simulink model "Simulation_Fahrmodell_v3"  (R2023b)
settings: Solver=ode14x  StartTime=0.0  StopTime=600  FixedStep=0.005  RelTol=1e-3
values from neighbouring files (symbols this model uses):
  bat = bat.computePack()    [DoE_main.m]    (also in DoE_main_sensitivity.m)
  cp = cp.computeP4Map(val_P4, 0, val_P4_DM, 0, 0)    [DoE_main.m]    (also in DoE_main_sensitivity.m = cp.computeP4Map(P4, E2, P4_DM, E3, E4))
  gb = gb.computeShiftMaps()    [DoE_main.m]    (also in DoE_main_sensitivity.m)
  P4 = cfgNum(cfg, 'P4', 0)    [DoE_main_sensitivity.m]    (also in PowertrainConfig.m = 0)
  P4_DM = cfgNum(cfg, 'P4_DM', 0)    [DoE_main_sensitivity.m]    (also in PowertrainConfig.m = 0)
  pt = pt.setupHybrid()    [DoE_main.m]    (also in DoE_main_sensitivity.m)
  veh = VehicleConfig()    [DoE_main.m]    (also in DoE_main_sensitivity.m)
undefined symbols (not defined in the file or in its folder): cp_Zelle_JpkgK, Ice_derfacLoadDecrease_MAP, Ice_derfacLoadIncrease_MAP, Ice_n_axis, Ice_relLoadMax_CUR_n, Ice_relLoadMax_CUR_val, Ice_rl_axis_norm, seconds, SKO_STREET_CHAL, SKO_WHEEL_TYP_CHAL, slip_pacejka, T_init_degC, Track, TT_sliced, use_turbo_model, v_Fzg_init_kmph
libraries: nesl_utility x15, fl_lib x9
(part 3 of 6)

== system Simulation_Fahrmodell_v3/Vehicle Dynamics Model /Drivetrain/Reifenmodell1/Schlupfberechnung ==
  S_BUS_IST_Profil_a : Inport
  S_BUS_IST_Profil_v : Inport  Port=2
  AND : Logic  AllPortsSameDT=off  OutDataTypeStr=boolean
  Abs1 : Abs  SaturateOnIntegerOverflow=off
  Add1 : Sum
  Constant : Constant
  Constant1 : Constant
  Constant2 : Constant  Value=150
  Delay One Step : Delay  DelayLength=1
  Gain : Gain  Gain=3.6
  Gain1 : Gain  Gain=1/100
  GreaterThan1 : RelationalOperator  Operator=>  OutDataTypeStr=boolean  RndMeth=Simplest  InputSameDT=off
  GreaterThan2 : RelationalOperator  Operator=<=  OutDataTypeStr=boolean  RndMeth=Simplest  InputSameDT=off
  PS-Simulink Converter : nesl_utility/PS-Simulink Converter  PhysicalDomain=network_engine_domain  SubClassName=ps_output  LeftPortType=input  RightPortType=output  PseudoPeriodic=off  Frequencies=[]  VectorFormat=inherit  Unit=inherit  AffineConversion=off
  PS-Simulink Converter15 : nesl_utility/PS-Simulink Converter  PhysicalDomain=network_engine_domain  SubClassName=ps_output  LeftPortType=input  RightPortType=output  PseudoPeriodic=off  Frequencies=[]  VectorFormat=inherit  Unit=inherit  AffineConversion=off
  Schlupf als f(a[m/s^2]) : fl_lib/Physical Signals/Lookup Tables/PS Lookup Table (1D)  x=[0 2 4 6 8 10 12]  f=[4 5 6.5 8.5 9.25 10 10]  interp_method=simscape.enum.interpolation.smooth  extrap_method=simscape.enum.extrapolation.nearest
  Schlupf als f(v[km/h]) : fl_lib/Physical Signals/Lookup Tables/PS Lookup Table (1D)  x=[0 20 40 60 80 100 120]  f=[6 5.9 5.5 5 4.5 4.1 4]  interp_method=simscape.enum.interpolation.smooth  extrap_method=simscape.enum.extrapolation.nearest
  Scope1 : Scope  NumInputPorts=5
  Scope4 : Scope  NumInputPorts=2
  Simulink-PS Converter : nesl_utility/Simulink-PS Converter  PhysicalDomain=network_engine_domain  SubClassName=ps_input  LeftPortType=input  RightPortType=output  PseudoPeriodic=off  Frequencies=[]  NoiseDistribution=none  NoiseParameters=[]  Unit=1  AffineConversion=off  FilteringAndDerivatives=provide  SimscapeFilterOrder=1  InputFilterTimeConstant=0.001  UdotUserProvided=0
  Simulink-PS Converter3 : nesl_utility/Simulink-PS Converter  PhysicalDomain=network_engine_domain  SubClassName=ps_input  LeftPortType=input  RightPortType=output  PseudoPeriodic=off  Frequencies=[]  NoiseDistribution=none  NoiseParameters=[]  Unit=1  AffineConversion=off  FilteringAndDerivatives=provide  SimscapeFilterOrder=1  InputFilterTimeConstant=0.001  UdotUserProvided=0
  Solver Configuration1 : nesl_utility/Solver Configuration  PhysicalDomain=network_engine_domain  SubClassName=solver  LeftPortType=input  RightPortType=generic  Tones=[]  Harmonics=[]  SimulateNoise=off  Profile=off  UseLocalSampling=off  EnableSwitchedLinearOptims=on  FrequencyDomain=off  UseCCode=off  RelTol=0.001  AbsTol=0.001  MinStep=1e-09  ToWorkspace=off  RevertToSquareIcSolve=off  NumHomotopyIterations=100  PhasorMode=off  PhasorModeNumHarmonics=1  ConsistencySolver=NEWTON_FTOL  CanonicalOrdering=UNORDERED  OptimizeIntermediates=UNOPTIMIZED  IndexReductionMethod=DerivativeReplacement  DoDC=off  ResidualTolerance=1e-09  ConsistencyTolSource=GLOBAL  ConsistencyAbsTol=0.001  ConsistencyRelTol=0.001  ConsistencyTolFactor=0.001  UseLocalSolver=off  LocalSolverChoice=NE_BACKWARD_EULER_ADVANCER  ResolveIndetEquations=on  FunctionEvalNumThread=1  LocalSolverSampleTime=0.001  DoFixedCost=off  MaxNonlinIter=3  MaxModeIter=2  ComputeImpulses=off  ImpulseIterations=2  LinearAlgebra=auto  LinearAlgebraNumThread=0  EquationFormulation=NE_TIME_EF  DelaysMemoryBudget=1024  AutomaticFiltering=on  FilteringTimeConstant=0.001  PartitionStorageMethod=AS_NEEDED  PartitionMemoryBudget=1024  PartitionMethod=ROBUST  MultibodyUseLocalSolver=off  MultibodyLocalSolverChoice=ODE1  MultibodyLocalSolverSampleTime=0.001
  Solver Configuration2 : nesl_utility/Solver Configuration  PhysicalDomain=network_engine_domain  SubClassName=solver  LeftPortType=input  RightPortType=generic  Tones=[]  Harmonics=[]  SimulateNoise=off  Profile=off  UseLocalSampling=off  EnableSwitchedLinearOptims=on  FrequencyDomain=off  UseCCode=off  RelTol=0.001  AbsTol=0.001  MinStep=1e-09  ToWorkspace=off  RevertToSquareIcSolve=off  NumHomotopyIterations=100  PhasorMode=off  PhasorModeNumHarmonics=1  ConsistencySolver=NEWTON_FTOL  CanonicalOrdering=UNORDERED  OptimizeIntermediates=UNOPTIMIZED  IndexReductionMethod=DerivativeReplacement  DoDC=off  ResidualTolerance=1e-09  ConsistencyTolSource=GLOBAL  ConsistencyAbsTol=0.001  ConsistencyRelTol=0.001  ConsistencyTolFactor=0.001  UseLocalSolver=off  LocalSolverChoice=NE_BACKWARD_EULER_ADVANCER  ResolveIndetEquations=on  FunctionEvalNumThread=1  LocalSolverSampleTime=0.001  DoFixedCost=off  MaxNonlinIter=3  MaxModeIter=2  ComputeImpulses=off  ImpulseIterations=2  LinearAlgebra=auto  LinearAlgebraNumThread=0  EquationFormulation=NE_TIME_EF  DelaysMemoryBudget=1024  AutomaticFiltering=on  FilteringTimeConstant=0.001  PartitionStorageMethod=AS_NEEDED  PartitionMemoryBudget=1024  PartitionMethod=ROBUST  MultibodyUseLocalSolver=off  MultibodyLocalSolverChoice=ODE1  MultibodyLocalSolverSampleTime=0.001
  Switch1 : Switch  Criteria=u2 > Threshold  SaturateOnIntegerOverflow=off  InputSameDT=off
  s max (%) : Outport
  s_fakt : Outport  Port=2
  wires:
  S_BUS_IST_Profil_a/1 -> Delay One Step/1
  GreaterThan1/1 -> AND/1  "abs(a) > 1 m/s^2"
  Constant1/1 -> GreaterThan1/2
  S_BUS_IST_Profil_v/1 -> Gain/1
  PS-Simulink Converter15/1 -> Scope1/2, Switch1/3  "s (v)"
  Gain1/1 -> Add1/1
  GreaterThan2/1 -> AND/2  "v <= 150 km/h"
  Delay One Step/1 -> Scope4/1, Abs1/1, Simulink-PS Converter/1
  Constant/1 -> Add1/2
  PS-Simulink Converter/1 -> Switch1/1, Scope1/1  "S a)"
  Gain/1 -> Simulink-PS Converter3/1, GreaterThan2/1  "v (km/h)"
  Add1/1 -> Scope1/5, s_fakt/1  "s_fakt"
  AND/1 -> Scope1/3, Switch1/2  "beide Bedingungen erfüllt"
  Switch1/1 -> Scope1/4, s max (%)/1, Gain1/1  "s max (%)"
  Constant2/1 -> GreaterThan2/2
  Abs1/1 -> GreaterThan1/1, Scope4/2
  connections:
  Schlupf als f(a[m/s^2])/LConn1 -- Solver Configuration1/RConn1 -- Simulink-PS Converter/RConn1
  PS-Simulink Converter/LConn1 -- Schlupf als f(a[m/s^2])/RConn1
  Simulink-PS Converter3/RConn1 -- Solver Configuration2/RConn1 -- Schlupf als f(v[km/h])/LConn1
  Schlupf als f(v[km/h])/RConn1 -- PS-Simulink Converter15/LConn1

== system Simulation_Fahrmodell_v3/Vehicle Dynamics Model /Driving Resistance/Subsystem/Fahrwiderstand1 ==
  note: Kraftfahrtechnisches Taschenbuch | SpringerLink
  note: Kraftfahrtechnisches Handbuch - Bosch 2024
  note: Massenfaktor: Multiplikationsfaktor zur Masse abh. Hubraum
  note: Luftwiderstand
  note: Geschwindigkeitswiderstand
  note: Rollwiderstand
  note: Steigungswiderstand
  X_BUS_CHAL : Inport
  BUS_STEIGUNG : Inport  Port=2
  F_x_N : Inport  Port=3
  Add : Sum  Inputs=++++
  Bus Selector1 : BusSelector  OutputSignals=S_BUS_EIG_RoWi_CHAL,S_BUS_EIG_GEW_CHAL,S_BUS_EIG_A_CHAL,S_BUS_EIG_Cw_CHAL,S_BUS_EIG_v_Bwert_CHAL
  Bus Selector4 : BusSelector  OutputSignals=M_BUS_EIG_CHAL
  Divide : Product  Inputs=*/
  Erdbeschleunigung : Gain  Gain=9.81
  Gain : Gain  Gain=0.5
  Gain{1..5} (5 alike) : Gain
  Integrator : Integrator  InitialCondition=0.01
  MATLAB Function : MATLAB Function  TreatAsAtomicUnit=on
  MATLAB Function1 : MATLAB Function  TreatAsAtomicUnit=on
  Math Function : Math  Operator=square
  Mux1 : Mux  Inputs=2
  Mux2 : Mux  Inputs=5
  Product : Product
  Product1 : Product  Inputs=5
  Product2 : Product
  Product8 : Product
  Roh Luft : Constant  Value=1.23
  Scope : Scope  NumInputPorts=2
  Scope2 : Scope  NumInputPorts=2
  Sum : Sum  Inputs=-+
  v : Outport
  wires:
  Bus Selector1/1 -> Gain1/1  "<S_BUS_EIG_RoWi_CHAL>"
  MATLAB Function/1(y) -> Product1/5  "cosd(alpha)"
  Math Function/1 -> Product1/4  "v ^ 2"
  MATLAB Function1/1(y) -> Product2/2  "sind(alpha)"
  BUS_STEIGUNG/1 -> MATLAB Function1/1(u), MATLAB Function/1(u)  "alpha"
  Bus Selector1/2 -> Gain2/1  "<S_BUS_EIG_GEW_CHAL>"
  Bus Selector1/3 -> Gain3/1  "<S_BUS_EIG_A_CHAL>"
  Erdbeschleunigung/1 -> Product2/1, Product/2  "m * g"
  Roh Luft/1 -> Gain/1  "rho"
  Product2/1 -> Add/4, Scope/1, Mux2/4  "Steigungswiderstand (N)"
  Integrator/1 -> v/1, Product8/2, Math Function/1  "v"
  Add/1 -> Scope/2, Mux1/2, Sum/1  "S_BUS_FLST_Wrls (N)"
  Mux2/1 -> Scope2/1
  Bus Selector1/5 -> Gain5/1  "<S_BUS_EIG_v_Bwert_CHAL>"
  Mux1/1 -> Scope2/2
  Bus Selector1/4 -> Gain4/1  "<S_BUS_EIG_Cw_CHAL>"
  Product1/1 -> Add/2, Mux2/2  "Luftwiderstand (N)"
  Product/1 -> Add/1, Mux2/1  "Rollwiderstand (N)"
  Gain/1 -> Product1/2  "0,5 * rho"
  Product8/1 -> Add/3, Mux2/3  "Geschwindigkeitswiderstand (N)"
  Bus Selector4/1 -> Bus Selector1/1  "<M_BUS_EIG_CHAL>"
  X_BUS_CHAL/1 -> Bus Selector4/1
  Gain1/1 -> Product/1  "f_R"
  Gain2/1 -> Erdbeschleunigung/1, Divide/2  "m"
  Gain3/1 -> Product1/1  "A"
  Gain4/1 -> Product1/3  "Cw"
  Gain5/1 -> Product8/1  "f_v"
  F_x_N/1 -> Sum/2  "F_x_N"
  Sum/1 -> Divide/1
  Divide/1 -> Integrator/1

== system Simulation_Fahrmodell_v3/Vehicle Dynamics Model /Drivetrain/Axle Load and Torque Distribution /Drive Topology Axle Load Distributor /Front Axle Load Calculator  ==
  M_Nm : Inport
  Achslast HA [%] : Inport  Port=2
  Display : Display
  Display1 : Display
  Display2 : Display
  Gain : Gain  Gain=0.01
  Radlast HA : Product
  Radlast HA [Nm] : Outport
  wires:
  Achslast HA [%]/1 -> Display/1, Gain/1
  M_Nm/1 -> Radlast HA/1
  Gain/1 -> Display1/1, Radlast HA/2
  Radlast HA/1 -> Display2/1, Radlast HA [Nm]/1

== system Simulation_Fahrmodell_v3/Vehicle Dynamics Model /Drivetrain/Axle Load and Torque Distribution /Drive Topology Axle Load Distributor /P4 AWD or AWD ==
  M_VA_Nm IN : Inport
  In3 : Inport  Port=2
  In2 : Inport  Port=3
  Switch : Switch  Criteria=u2 > Threshold  SaturateOnIntegerOverflow=off  InputSameDT=off
  Out1 : Outport
  wires:
  In3/1 -> Switch/3
  Switch/1 -> Out1/1
  M_VA_Nm IN/1 -> Switch/1
  In2/1 -> Switch/2

== system Simulation_Fahrmodell_v3/Vehicle Dynamics Model /Drivetrain/Axle Load and Torque Distribution /Drive Topology Axle Load Distributor /P4 AWD or AWD1 ==
  In2 : Inport
  M_VA_Nm IN : Inport  Port=2
  In3 : Inport  Port=3
  Switch : Switch  Criteria=u2 > Threshold  SaturateOnIntegerOverflow=off  InputSameDT=off
  Out1 : Outport
  wires:
  In2/1 -> Switch/2
  M_VA_Nm IN/1 -> Switch/1
  Switch/1 -> Out1/1
  In3/1 -> Switch/3

== system Simulation_Fahrmodell_v3/Vehicle Dynamics Model /Drivetrain/Axle Load and Torque Distribution /Drive Topology Axle Load Distributor /Rear Axle Load Calculator  ==
  M_Nm : Inport
  Achslast VA [%] : Inport  Port=2
  Gain : Gain  Gain=0.01
  Radlast VA : Product
  Radlast VA [Nm] : Outport
  wires:
  Achslast VA [%]/1 -> Gain/1
  M_Nm/1 -> Radlast VA/1
  Radlast VA/1 -> Radlast VA [Nm]/1
  Gain/1 -> Radlast VA/2

== system Simulation_Fahrmodell_v3/Vehicle Dynamics Model /Drivetrain/GETRIEBE auswahl VK, EV/Transmission Selector/ EV Single-Speed ==
  n_mot_Upmin : Inport
  i_AG : Inport  Port=2
  "Gaspedalposition [0, 1]" : Inport  Port=3
  Constant : Constant  Value=gb.i_GET_EV
  "GET -> AG" : Product
  Terminator : Terminator
  Terminator1 : Terminator
  i_GES : Outport
  i_GES_delay : Outport  Port=2
  wires:
  "GET -> AG"/1 -> i_GES_delay/1, i_GES/1  "i_GES"
  Constant/1 -> "GET -> AG"/2
  i_AG/1 -> "GET -> AG"/1  "i_AG"
  n_mot_Upmin/1 -> Terminator/1
  "Gaspedalposition [0, 1]"/1 -> Terminator1/1

== system Simulation_Fahrmodell_v3/Vehicle Dynamics Model /Drivetrain/GETRIEBE auswahl VK, EV/Transmission Selector/ICE Multi-Speed ==
  note: Determination of minimum and maximum speed depending on accelerator pedal position and actual gear
  n_mot_Upmin : Inport
  i_AG : Inport  Port=2
  "Gaspedalposition [0, 1]" : Inport  Port=3
  Aktueller Gang : Gain
  Begrenzung Gang : Saturate  UpperLimit=10  LowerLimit=1
  Bus Creator : BusCreator  Inputs=3
  Delay Aktueller Gang Init: 1 : Delay  DelayLength=1  InitialCondition=1
  Delay Aktueller Gang Init: 2 : Delay  DelayLength=1  InitialConditionSource=Input port  InitialCondition=1
      settings: InputPortMap=u0,p4
  Ermittlung min und max Drehzahl abh. Gaspedalposition und Ist-Gang : Subsystem
  "GET -> AG" : Product
  Gain1 : Gain
  "Gang -> i_GET Generic 1" : Lookup_n-D  NumberOfTableDimensions=1  BreakpointsForDimension1=[1:1:gb.No_Gears]  Table=gb.Gear_Ratio  InternalRulePriority=Speed  RndMeth=Simplest
  Init: i_GES(1) Generic 1 : Constant  Value=5*3.204
  Scope : Scope  NumInputPorts=3
  Simulation Doppelkupplung (Gangwechsel ohne Zugkraftunterbrechung) orig2 : Subsystem
  Subsystem1 : Subsystem
  i_GES : Outport
  i_GES_delay : Outport  Port=2
  wires:
  Subsystem1/1(Current_Gear) -> Begrenzung Gang/1
  Init: i_GES(1) Generic 1/1 -> Delay Aktueller Gang Init: 2/2
  Ermittlung min und max Drehzahl abh. Gaspedalposition und Ist-Gang/2(n_min_Upmin) -> Subsystem1/3(downshift), Bus Creator/2
  Bus Creator/1 -> Scope/1
  Ermittlung min und max Drehzahl abh. Gaspedalposition und Ist-Gang/1(n_max_Upmin) -> Subsystem1/2(upshift), Bus Creator/3
  Gain1/1 -> "GET -> AG"/1  "i_AG"
  "Gang -> i_GET Generic 1"/1 -> "GET -> AG"/2
  "Gaspedalposition [0, 1]"/1 -> Ermittlung min und max Drehzahl abh. Gaspedalposition und Ist-Gang/1(Gaspedalposition)
  Simulation Doppelkupplung (Gangwechsel ohne Zugkraftunterbrechung) orig2/1(i_GET DKG) -> i_GES/1, Delay Aktueller Gang Init: 2/1, Scope/2
  n_mot_Upmin/1 -> Subsystem1/1(Current rpm), Bus Creator/1  "n_mot_Upmin"
  Begrenzung Gang/1 -> Delay Aktueller Gang Init: 1/1, Aktueller Gang/1
  Delay Aktueller Gang Init: 1/1 -> Ermittlung min und max Drehzahl abh. Gaspedalposition und Ist-Gang/2(Gang)
  i_AG/1 -> Gain1/1
  Aktueller Gang/1 -> "Gang -> i_GET Generic 1"/1, Simulation Doppelkupplung (Gangwechsel ohne Zugkraftunterbrechung) orig2/2(GANG), Scope/3  "GANG"
  "GET -> AG"/1 -> Simulation Doppelkupplung (Gangwechsel ohne Zugkraftunterbrechung) orig2/1(i_GET)  "i_GES"
  Delay Aktueller Gang Init: 2/1 -> i_GES_delay/1

== system Simulation_Fahrmodell_v3/Vehicle Dynamics Model /Drivetrain/Operating Strategy 1.1/EMs Priority (Ep)/SOC LIMIT ==
  tq_wheel_ICE_des_Ep : Inport
  SOC : Inport  Port=2
  tq_wheel_Elec_des_Ep : Inport  Port=3
  Add : Sum
  Constant : Constant  Value=0
  Ep_SOC Limit : Constant  Value=20
  Relational Operator : RelationalOperator  Operator=>  OutDataTypeStr=boolean  RndMeth=Simplest  InputSameDT=off
  Switch : Switch  Criteria=u2 > Threshold  SaturateOnIntegerOverflow=off  InputSameDT=off
  Switch1 : Switch  Criteria=u2 > Threshold  SaturateOnIntegerOverflow=off  InputSameDT=off
  "tq_wheel_ICE_des_Ep " : Outport
  "tq_wheel_Elec_des_Ep " : Outport  Port=2
  wires:
  Ep_SOC Limit/1 -> Relational Operator/2
  Relational Operator/1 -> Switch1/2, Switch/2
  tq_wheel_Elec_des_Ep/1 -> Switch1/1, Add/2
  Switch1/1 -> "tq_wheel_Elec_des_Ep "/1
  SOC/1 -> Relational Operator/1
  Constant/1 -> Switch1/3
  tq_wheel_ICE_des_Ep/1 -> Add/1, Switch/1
  Switch/1 -> "tq_wheel_ICE_des_Ep "/1
  Add/1 -> Switch/3

== system Simulation_Fahrmodell_v3/Vehicle Dynamics Model /Drivetrain/Operating Strategy 1.1/Wheel-to-Shaft Converter and Demand Validators /EV Primary Axle Torque Path Selector ==
  tq_wheel_Primary_axle_des : Inport
  " " : Constant  Value=veh.EV
  "  " : Constant  Value=0
  "   " : Constant  Value=pt.E3
  "    " : Constant  Value=pt.E4
  "       " : Constant  Value=pt.E2
  Constant5 : Constant  Value=veh.MainAxle_TorqueSplit_int
  OR1 : Logic  Operator=OR  Inputs=3  IconShape=distinctive  AllPortsSameDT=off  OutDataTypeStr=boolean
  Product1 : Product
  Switch : Switch  Criteria=u2 > Threshold  SaturateOnIntegerOverflow=off  InputSameDT=off
  Switch3 : Switch  Criteria=u2 > Threshold  SaturateOnIntegerOverflow=off  InputSameDT=off
  tq_wheel_EV_des : Outport
  wires:
  "   "/1 -> OR1/2
  OR1/1 -> Switch3/2
  "  "/1 -> Switch/3
  " "/1 -> Switch/2
  Switch/1 -> Switch3/3, Product1/1
  Product1/1 -> Switch3/1
  Constant5/1 -> Product1/2
  "       "/1 -> OR1/1
  "    "/1 -> OR1/3
  Switch3/1 -> tq_wheel_EV_des/1
  tq_wheel_Primary_axle_des/1 -> Switch/1

== system Simulation_Fahrmodell_v3/Vehicle Dynamics Model /Drivetrain/Operating Strategy 1.1/Wheel-to-Shaft Converter and Demand Validators /Secondary Axle Torque Path Selector ==
  tq_wheel_Primary_axle_des : Inport
  tq_wheel_Secondary_axle_des : Inport  Port=2
  "  " : Constant  Value=pt.E4
  "   " : Constant
  "    " : Constant  Value=pt.E3
  "         " : Constant  Value=0
  "              " : Constant  Value=pt.E2
  Add : Sum  Inputs=+-
  Constant2 : Constant  Value=veh.MainAxle_TorqueSplit_int
  Constant3 : Constant  Value=pt.P4
  Constant4 : Constant  Value=pt.P4_DM
  OR : Logic  Operator=OR  Inputs=3  IconShape=distinctive  AllPortsSameDT=off  OutDataTypeStr=boolean
  OR1 : Logic  Operator=OR  IconShape=distinctive  AllPortsSameDT=off  OutDataTypeStr=boolean
  Product : Product
  Switch1 : Switch  Criteria=u2 > Threshold  SaturateOnIntegerOverflow=off  InputSameDT=off
  Switch2 : Switch  Criteria=u2 > Threshold  SaturateOnIntegerOverflow=off  InputSameDT=off
  tq_wheel_P4_des : Outport
  wires:
  "  "/1 -> OR/3
  "   "/1 -> Add/1
  "         "/1 -> Switch2/3
  OR/1 -> Switch1/2
  tq_wheel_Primary_axle_des/1 -> Product/1
  Product/1 -> Switch1/1
  "              "/1 -> OR/1
  Constant2/1 -> Add/2
  OR1/1 -> Switch2/2
  "    "/1 -> OR/2
  Switch2/1 -> Switch1/3
  Add/1 -> Product/2
  Switch1/1 -> tq_wheel_P4_des/1  "tq_wheel_P4_des"
  tq_wheel_Secondary_axle_des/1 -> Switch2/1
  Constant4/1 -> OR1/2
  Constant3/1 -> OR1/1

== system Simulation_Fahrmodell_v3/Vehicle Dynamics Model /Drivetrain/Primary and Secondary Axle Powertrain Selector/Primary Axle Powertrain Selector/Electric Drive ==
  Regelfaktor : Inport
  n_mot_Upmin : Inport  Port=2
  i_ges : Inport  Port=3
  iAG : Inport  Port=4
  Torque_sh : Inport  Port=5
  Variant Subsystem : Subsystem  Variant=on
  Tq_Primary_axle : Outport
  wires:
  iAG/1 -> Variant Subsystem/3(iAG)
  i_ges/1 -> Variant Subsystem/1(i_ges)  "i_GES"
  n_mot_Upmin/1 -> Variant Subsystem/4(n_mot_Upmin)  "Motordrehzahl (1/min)"
  Regelfaktor/1 -> Variant Subsystem/2(Regelfaktor1)
  Variant Subsystem/1("M_Nm GET VKM, EM, P1, P2, P3") -> Tq_Primary_axle/1
  Torque_sh/1 -> Variant Subsystem/5(Torque_sh)

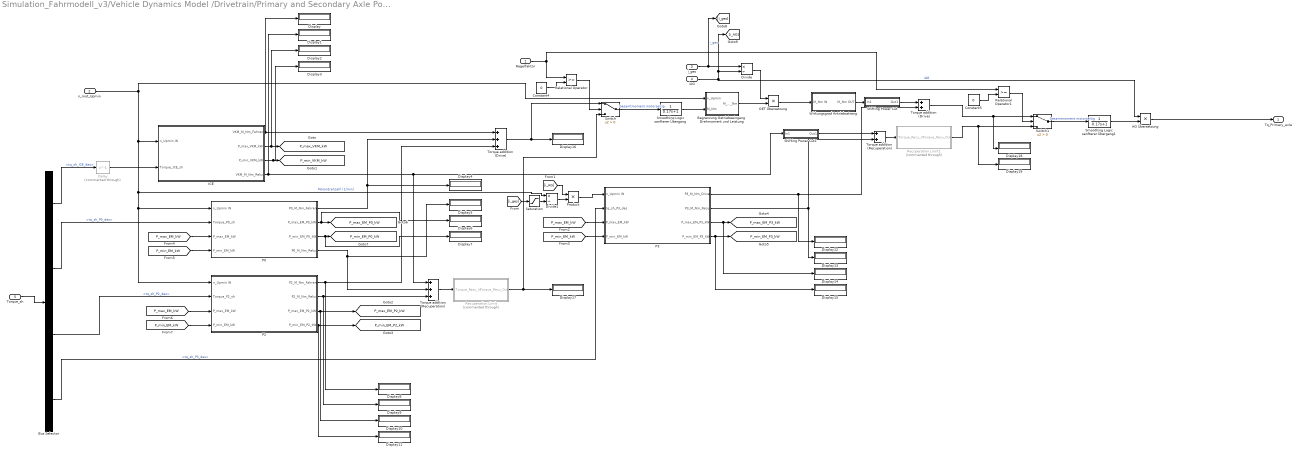
== system Simulation_Fahrmodell_v3/Vehicle Dynamics Model /Drivetrain/Primary and Secondary Axle Powertrain Selector/Primary Axle Powertrain Selector/Hybrid Drive ==
  Regelfaktor : Inport
  n_mot_Upmin : Inport  Port=2
  i_ges : Inport  Port=3
  iAG : Inport  Port=4
  Torque_sh : Inport  Port=5
  AG Übersetzung : Product
  Begrenzung Getriebeeingang Drehmoment und Leistung : Subsystem
  Bus Selector : BusSelector  OutputSignals=tq_sh_ICE_des,tq_sh_P0_des,tq_sh_P2_des,tq_sh_P3_des
  Constant4 : Constant  Value=0
  Constant5 : Constant  Value=0
  Delay : Delay  Commented=through  DelayLength=1  InputProcessing=Columns as channels (frame based)
  Display{,1..19} (20 alike) : Display
  Divide : Product  Inputs=*/
  Divide1 : Product  Inputs=*/
  GET Übersetzung : Product
  ICE : Subsystem  VariantControl=true
  P0 : Subsystem  Variant=on
  P2 : Subsystem  Variant=on
  P3 : Subsystem  Variant=on
  Product : Product
  Recuperation Limit : Subsystem  Commented=through
  Recuperation Limit1 : Subsystem  Commented=through
  Relational Operator : RelationalOperator  OutDataTypeStr=boolean  RndMeth=Simplest  InputSameDT=off
  Relational Operator1 : RelationalOperator  OutDataTypeStr=boolean  RndMeth=Simplest  InputSameDT=off
  Saturation : Saturate  UpperLimit=inf  LowerLimit=1
  Shifting Power Cut : Subsystem
  Shifting Power Cut1 : Subsystem
  Smoothing Logic sanfterer Übergang : TransferFcn  Denominator=[0.17 1]
  Smoothing Logic sanfterer Übergang1 : TransferFcn  Denominator=[0.17 1]
  Switch : Switch  Criteria=u2 > Threshold  SaturateOnIntegerOverflow=off  InputSameDT=off
  Switch1 : Switch  Criteria=u2 > Threshold  SaturateOnIntegerOverflow=off  InputSameDT=off
  Torque addition (Drive) : Sum
  "Torque addition (Drive) " : Sum  Inputs=+++
  Torque addition (Recuperation) : Sum
  "Torque addition (Recuperation) " : Sum  Inputs=+++
  Wirkungsgrad Antriebsstrang : Subsystem
  Tq_Primary_axle : Outport
  tag scope: P_max_EM_P0_kW=global, P_max_EM_P2_kW=global, P_max_EM_P3_kW=global, P_max_VKM_kW=global, P_min_EM_P0_kW=global, P_min_EM_P2_kW=global, P_min_EM_P3_kW=global, P_min_VKM_kW=global
  wires:
  iAG/1 -> Divide/2, [i_AG], AG Übersetzung/1  "iAG"
  i_ges/1 -> [i_ges], Divide/1  "i_ges"
  Switch/1 -> Smoothing Logic sanfterer Übergang/1  "Gesamtmoment motorseitig"
  Begrenzung Getriebeeingang Drehmoment und Leistung/1(M_begr_Nm) -> GET Übersetzung/2
  Constant4/1 -> Relational Operator/2
  Smoothing Logic sanfterer Übergang/1 -> Begrenzung Getriebeeingang Drehmoment und Leistung/2(M_Nm)
  P3/1(P3_M_Nm_Drive) -> Display12/1, Torque addition (Drive)/2
  "Torque addition (Drive) "/1 -> Switch/1, Display16/1
  GET Übersetzung/1 -> Wirkungsgrad Antriebsstrang/1(M_Nm IN)
  P2/1(P2_M_Nm_Fahren) -> Display8/1, "Torque addition (Drive) "/3
  Constant5/1 -> Relational Operator1/2
  P2/2(P2_M_Nm_Reku) -> Display9/1, "Torque addition (Recuperation) "/3
  P3/2(P3_M_Nm_Recu) -> Display13/1, Torque addition (Recuperation)/2
  Smoothing Logic sanfterer Übergang1/1 -> AG Übersetzung/2
  Regelfaktor/1 -> Relational Operator1/1, Relational Operator/1
  Divide/1 -> GET Übersetzung/1
  AG Übersetzung/1 -> Tq_Primary_axle/1
  Relational Operator1/1 -> Switch1/2
  Relational Operator/1 -> Switch/2
  Wirkungsgrad Antriebsstrang/1(M_Nm OUT) -> Shifting Power Cut/1(In1)
  Switch1/1 -> Smoothing Logic sanfterer Übergang1/1  "Gesamtmoment motorseitig"
  Torque addition (Drive)/1 -> Display18/1, Switch1/1
  P0/1(P0_M_Nm_Fahren) -> Display4/1, "Torque addition (Drive) "/2
  n_mot_Upmin/1 -> Divide1/1, P2/1(n_Upmin IN), P0/1(n_Upmin IN), ICE/1(n_Upmin IN), Begrenzung Getriebeeingang Drehmoment und Leistung/1(n_Upmin)  "Motordrehzahl (1/min)"
  ICE/1(VKM_M_Nm_Fahren) -> "Torque addition (Drive) "/1, Display/1
  ICE/4(VKM_M_Nm_Reku) -> Display1/1, "Torque addition (Recuperation) "/1, Shifting Power Cut1/1(In1)
  ICE/2(P_max_VKM_kW) -> Display2/1, [P_max_VKM_kW]
  ICE/3(P_min_VKM_kW) -> Display3/1, [P_min_VKM_kW]
  [P_max_EM_kW] -> P2/3(P_max_EM_kW)
  [P_min_EM_kW] -> P2/4(P_min_EM_kW)
  P2/3(P_max_EM_P2_kW) -> Display10/1, [P_max_EM_P2_kW]
  P2/4(P_min_EM_P2_kW) -> Display11/1, [P_min_EM_P2_kW]
  [P_max_EM_kW] -> P0/3(P_max_EM_kW)
  [P_min_EM_kW] -> P0/4(P_min_EM_kW)
  P0/2(P_max_EM_P0_kW) -> Display6/1, [P_max_EM_P0_kW]
  P0/3(P_min_EM_P0_kW) -> Display7/1, [P_min_EM_P0_kW]
  P0/4(P0_M_Nm_Reku) -> Display5/1, "Torque addition (Recuperation) "/2
  P3/3(P_max_EM_P3_kW) -> Display14/1, [P_max_EM_P3_kW]
  P3/4(P_min_EM_P3_kW) -> Display15/1, [P_min_EM_P3_kW]
  [P_max_EM_kW] -> P3/3(P_max_EM_kW)
  [P_min_EM_kW] -> P3/4(P_min_EM_kW)
  Torque addition (Recuperation)/1 -> Recuperation Limit1/1(Torque_Recu_In)
  Torque_sh/1 -> Bus Selector/1
  Bus Selector/1 -> Delay/1  "<tq_sh_ICE_des>"
  Bus Selector/2 -> P0/2(Torque_P0_sh)  "<tq_sh_P0_des>"
  Bus Selector/3 -> P2/2(Torque_P2_sh)  "<tq_sh_P2_des>"
  Bus Selector/4 -> P3/2(tq_sh_P3_des)  "<tq_sh_P3_des>"
  Divide1/1 -> Product/2
  [i_ges] -> Saturation/1
  [i_AG] -> Product/1
  Product/1 -> P3/1(n_Upmin IN)
  Saturation/1 -> Divide1/2
  Recuperation Limit/1(Torque_Recu_Out) -> Switch/3, Display17/1
  "Torque addition (Recuperation) "/1 -> Recuperation Limit/1(Torque_Recu_In)
  Recuperation Limit1/1(Torque_Recu_Out) -> Display19/1, Switch1/3
  Delay/1 -> ICE/2(Torque_ICE_sh)
  Shifting Power Cut/1(Out1) -> Torque addition (Drive)/1
  Shifting Power Cut1/1(Out1) -> Torque addition (Recuperation)/1

== system Simulation_Fahrmodell_v3/Vehicle Dynamics Model /Drivetrain/Primary and Secondary Axle Powertrain Selector/Secondary Axle Powertrain Selector/Auswahl P4, P4_Dual-Motor ==
  note: 1) Add Subsystem or Model blocks as valid variant choices.
      | 2) You cannot connect blocks at this level. At simulation, connectivity is automatically
      | determined, based on the active variant and port name matching.
  n_mot_Upmin : Inport
  Regelfaktor1 : Inport  Port=2
  iAG : Inport  Port=3
  i_ges : Inport  Port=4
  Torque_sh : Inport  Port=5
  No Secondary Axle : Subsystem  VariantControl=pt.P4_DM == 0 && pt.P4 == 0
  P4 / E2 Single Motor : Subsystem  VariantControl=pt.P4 == 1
  P4 / E3 / E4 Dual Motor : Subsystem  VariantControl=pt.P4_DM == 1
  M_Nm GET P4 : Outport

== system Simulation_Fahrmodell_v3/Vehicle Dynamics Model /Drivetrain/GETRIEBE auswahl VK, EV/Transmission Selector/ICE Multi-Speed/Ermittlung min und max Drehzahl abh. Gaspedalposition und Ist-Gang ==
  Gaspedalposition : Inport
  Gang : Inport  Port=2
  Kennfeld n_max_Upmin : Lookup_n-D  BreakpointsForDimension1=gb.pedal_pos  BreakpointsForDimension2=gb.Gears  Table=gb.n_max_Upmin  InternalRulePriority=Speed  RndMeth=Simplest
      settings: InputPortMap=u0,u1
  Kennfeld n_min_Upmin : Lookup_n-D  BreakpointsForDimension1=gb.pedal_pos  BreakpointsForDimension2=gb.Gears  Table=gb.n_min_Upmin  InternalRulePriority=Speed  RndMeth=Simplest
      settings: InputPortMap=u0,u1
  n_max_Upmin : Outport
  n_min_Upmin : Outport  Port=2
  wires:
  Kennfeld n_min_Upmin/1 -> n_min_Upmin/1  "n_min_Upmin"
  Gaspedalposition/1 -> Kennfeld n_min_Upmin/1, Kennfeld n_max_Upmin/1
  Gang/1 -> Kennfeld n_max_Upmin/2, Kennfeld n_min_Upmin/2
  Kennfeld n_max_Upmin/1 -> n_max_Upmin/1  "n_max_Upmin"

== system Simulation_Fahrmodell_v3/Vehicle Dynamics Model /Drivetrain/GETRIEBE auswahl VK, EV/Transmission Selector/ICE Multi-Speed/Simulation Doppelkupplung (Gangwechsel ohne Zugkraftunterbrechung) orig2 ==
  i_GET : Inport
  GANG : Inport  Port=2
  Add : Sum
  Berechne prozentuale Zeit bis zum 0.3s : Product  Inputs=*/
  Berechne Negation der prozentualen Zeit : Sum  Inputs=+-
  Berechnung Zeit : Integrator  ExternalReset=falling
  Clock : Clock
  Constant : Constant  Value=0
  Constant1 : Constant
  Delay : Delay  DelayLength=1
  Display5 : Display
  Gang davor * proz. Zeit : Product
  Gang neu * proz. Zeit : Product
  "Nach Trigger -> 0.3s auf True halten" : MATLAB Function  TreatAsAtomicUnit=on
  "Prozentuale Zeit = 0 -> kein Gangwechsel" : RelationalOperator  Operator===  OutDataTypeStr=boolean  RndMeth=Simplest  InputSameDT=off
  Scope : Scope  NumInputPorts=2
  Scope1 : Scope
  Scope2 : Scope  NumInputPorts=2
  Switch : Switch  Criteria=u2 > Threshold  SaturateOnIntegerOverflow=off  InputSameDT=off
  Time to hold (s) : Constant  Value=0.15
  Vgl. Gang aktuell und Gang davor : RelationalOperator  Operator=~=  OutDataTypeStr=boolean  RndMeth=Simplest  InputSameDT=off
  Vorheriger Wert : Subsystem
  Zappeln vermeiden : Delay  DelayLength=1
  i_GET DKG : Outport
  wires:
  "Prozentuale Zeit = 0 -> kein Gangwechsel"/1 -> Switch/2
  Switch/1 -> i_GET DKG/1
  Constant/1 -> "Prozentuale Zeit = 0 -> kein Gangwechsel"/2
  Gang davor * proz. Zeit/1 -> Add/1
  Berechnung Zeit/1 -> Berechne prozentuale Zeit bis zum 0.3s/1
  Berechne Negation der prozentualen Zeit/1 -> Gang davor * proz. Zeit/2
  Add/1 -> Switch/3
  Vgl. Gang aktuell und Gang davor/1 -> "Nach Trigger -> 0.3s auf True halten"/2(enableSignal)
  Delay/1 -> Vgl. Gang aktuell und Gang davor/2
  Constant1/1 -> Berechne Negation der prozentualen Zeit/1
  "Nach Trigger -> 0.3s auf True halten"/1(out) -> Display5/1, Berechnung Zeit/1, Berechnung Zeit/2, Scope/2  "Output"
  Vorheriger Wert/1(Out1) -> Scope2/1, Gang davor * proz. Zeit/1
  Gang neu * proz. Zeit/1 -> Add/2
  Clock/1 -> "Nach Trigger -> 0.3s auf True halten"/1(clkTime)
  Zappeln vermeiden/1 -> Switch/1
  Berechne prozentuale Zeit bis zum 0.3s/1 -> Scope1/1, Gang neu * proz. Zeit/2, "Prozentuale Zeit = 0 -> kein Gangwechsel"/1, Berechne Negation der prozentualen Zeit/2
  i_GET/1 -> Scope2/2, Gang neu * proz. Zeit/1, Zappeln vermeiden/1, Vorheriger Wert/1(In1)
  Time to hold (s)/1 -> "Nach Trigger -> 0.3s auf True halten"/3(timeWait), Berechne prozentuale Zeit bis zum 0.3s/2
  GANG/1 -> Delay/1, Scope/1, Vgl. Gang aktuell und Gang davor/1

== system Simulation_Fahrmodell_v3/Vehicle Dynamics Model /Drivetrain/GETRIEBE auswahl VK, EV/Transmission Selector/ICE Multi-Speed/Subsystem1 ==
  Current rpm : Inport
  upshift : Inport  Port=2
  downshift : Inport  Port=3
  Begrenzung Gang1 : Saturate  UpperLimit=10  LowerLimit=1
  Constant : Constant  Value=0.005
  Constant3 : Constant  Value=gb.shiftDelay
  Delay : Delay  DelayLength=1
  "Desired Gear " : Subsystem
  "Locktime Bypass Conditions " : Subsystem
  Relational Operator3 : RelationalOperator  Operator=<=  OutDataTypeStr=boolean  RndMeth=Simplest  InputSameDT=off
  Relational Operator4 : RelationalOperator  OutDataTypeStr=boolean  RndMeth=Simplest  InputSameDT=off
  "Shift Delay and Clutch Disengagement " : MATLAB Function  TreatAsAtomicUnit=on
  gear latch : MATLAB Function  TreatAsAtomicUnit=on
  Current_Gear : Outport
  tag scope: Clutch_Engaged=global
  wires:
  Relational Operator4/1 -> "Desired Gear "/2(Upshift_Signal), gear latch/1(upshift)  "u"
  "Shift Delay and Clutch Disengagement "/1(currentGear) -> Begrenzung Gang1/1  "Normal"
  Constant/1 -> "Shift Delay and Clutch Disengagement "/2(dt)
  Begrenzung Gang1/1 -> Current_Gear/1, Delay/1  "Normal"
  "Shift Delay and Clutch Disengagement "/2(clutchEngaged) -> [Clutch_Engaged]
  Constant3/1 -> "Shift Delay and Clutch Disengagement "/3(shiftDelay)
  Relational Operator3/1 -> gear latch/2(downshift), "Desired Gear "/4(Downshift_Signal)  "d"
  Current rpm/1 -> Relational Operator3/1, "Locktime Bypass Conditions "/2(Current Rpm), Relational Operator4/1  "Current Rpm"
  upshift/1 -> Relational Operator4/2, "Locktime Bypass Conditions "/1(Gear upshift Rpm)  "Gear upshift Rpm"
  downshift/1 -> Relational Operator3/2, "Locktime Bypass Conditions "/3(Gear downshift Rpm)  "Gear downshift Rpm"
  "Locktime Bypass Conditions "/1(cmd_Bypass_Lock_time) -> gear latch/3(cmd_Bypass_Lock_time)  "bypass"
  Delay/1 -> "Desired Gear "/1(Current Gear)
  gear latch/1(shift_cmd) -> "Desired Gear "/3(cmd)  "cmd"
  "Desired Gear "/1(desiredGear) -> "Shift Delay and Clutch Disengagement "/1(desiredGear)

== system Simulation_Fahrmodell_v3/Vehicle Dynamics Model /Drivetrain/Primary and Secondary Axle Powertrain Selector/Primary Axle Powertrain Selector/Electric Drive/Variant Subsystem ==
  note: 1) Add Subsystem or Model blocks as valid variant choices.
      | 2) You cannot connect blocks at this level. At simulation, connectivity is automatically
      | determined, based on the active variant and port name matching.
  i_ges : Inport
  Regelfaktor1 : Inport  Port=2
  iAG : Inport  Port=3
  n_mot_Upmin : Inport  Port=4
  Torque_sh : Inport  Port=5
  EV Dual Motor : Subsystem  VariantControl=pt.E1 == 1
  EV Single Motor : Subsystem  VariantControl=pt.E0 == 1
  "M_Nm GET VKM, EM, P1, P2, P3" : Outport

== system Simulation_Fahrmodell_v3/Vehicle Dynamics Model /Drivetrain/Primary and Secondary Axle Powertrain Selector/Primary Axle Powertrain Selector/Hybrid Drive/Begrenzung Getriebeeingang Drehmoment und Leistung ==
  n_Upmin : Inport
  M_Nm : Inport  Port=2
  Abs : Abs  SaturateOnIntegerOverflow=off
  Begrenzung Drehmoment : Constant  Value=8250
  Begrenzung Leistung : Constant  Value=470
  Constant : Constant
  Constant1 : Constant  Value=2*pi/60/1000
  Divide : Product  Inputs=*//
  Gain : Gain  Gain=-1
  Max1 : MinMax  Inputs=3
  Max2 : MinMax  Function=max  Inputs=2
  Switch : Switch  Criteria=u2 > Threshold  SaturateOnIntegerOverflow=off  InputSameDT=off
  Switch1 : Switch  Criteria=u2 > Threshold  SaturateOnIntegerOverflow=off  InputSameDT=off
  M_begr_Nm : Outport
  wires:
  n_Upmin/1 -> Max2/1
  Begrenzung Leistung/1 -> Divide/1  "P_begr_Nm"
  Constant1/1 -> Divide/2
  Constant/1 -> Max2/2
  Max2/1 -> Divide/3
  Divide/1 -> Max1/3
  Begrenzung Drehmoment/1 -> Max1/2
  Switch/1 -> Max1/1
  Switch1/1 -> M_begr_Nm/1
  M_Nm/1 -> Switch1/2, Switch/2, Switch/1, Abs/1
  Abs/1 -> Switch/3
  Max1/1 -> Gain/1, Switch1/1
  Gain/1 -> Switch1/3

== system Simulation_Fahrmodell_v3/Vehicle Dynamics Model /Drivetrain/Primary and Secondary Axle Powertrain Selector/Primary Axle Powertrain Selector/Hybrid Drive/ICE ==
  n_Upmin IN : Inport
  Torque_ICE_sh : Inport  Port=2
  Berechnung Leistung 1 : Subsystem
  Berechnung Leistung 4 : Subsystem
  Constant : Constant  Value=-25
  "Max. Kennlinie VKM, Fahren" : Lookup_n-D  NumberOfTableDimensions=1  BreakpointsForDimension1=cp.speed_breakpoints_ICE  Table=cp.torque_values_ICE  InternalRulePriority=Speed  RndMeth=Simplest
  Min : MinMax  Inputs=2
  Saturation : Saturate  UpperLimit=1000  LowerLimit=0
  Turbo Lag (Beta) : Subsystem  Commented=on
  VKM_M_Nm_Fahren : Outport
  P_max_VKM_kW : Outport  Port=2
  P_min_VKM_kW : Outport  Port=3
  VKM_M_Nm_Reku : Outport  Port=4
  tag scope: tq_sh_ICE_max=global
  wires:
  n_Upmin IN/1 -> Berechnung Leistung 1/1(n_Upmin), Berechnung Leistung 4/1(n_Upmin), "Max. Kennlinie VKM, Fahren"/1  "Motordrehzahl (1/min)"
  "Max. Kennlinie VKM, Fahren"/1 -> [tq_sh_ICE_max], Min/1  "Torque_ICE_Limit"
  Torque_ICE_sh/1 -> Saturation/1
  Constant/1 -> VKM_M_Nm_Reku/1, Berechnung Leistung 4/2(M_Nm)  "VKM_M_Nm_Reku"
  Saturation/1 -> Min/2
  Min/1 -> VKM_M_Nm_Fahren/1, Berechnung Leistung 1/2(M_Nm)  "VKM_M_Nm_Fahren"
  Berechnung Leistung 1/1(P_kW) -> P_max_VKM_kW/1
  Berechnung Leistung 4/1(P_kW) -> P_min_VKM_kW/1

== system Simulation_Fahrmodell_v3/Vehicle Dynamics Model /Drivetrain/Primary and Secondary Axle Powertrain Selector/Primary Axle Powertrain Selector/Hybrid Drive/P0 ==
  note: 1) Add Subsystem or Model blocks as valid variant choices.
      | 2) You cannot connect blocks at this level. At simulation, connectivity is automatically
      | determined, based on the active variant and port name matching.
  n_Upmin IN : Inport
  Torque_P0_sh : Inport  Port=2
  P_max_EM_kW : Inport  Port=3
  P_min_EM_kW : Inport  Port=4
  P0 Motor : Subsystem  VariantControl=pt.P0 == 1
  P0 Motor disabled : Subsystem  VariantControl=pt.P0 == 0
  P0_M_Nm_Fahren : Outport
  P_max_EM_P0_kW : Outport  Port=2
  P_min_EM_P0_kW : Outport  Port=3
  P0_M_Nm_Reku : Outport  Port=4

== system Simulation_Fahrmodell_v3/Vehicle Dynamics Model /Drivetrain/Primary and Secondary Axle Powertrain Selector/Primary Axle Powertrain Selector/Hybrid Drive/P2 ==
  note: 1) Add Subsystem or Model blocks as valid variant choices.
      | 2) You cannot connect blocks at this level. At simulation, connectivity is automatically
      | determined, based on the active variant and port name matching.
  n_Upmin IN : Inport
  Torque_P2_sh : Inport  Port=2
  P_max_EM_kW : Inport  Port=3
  P_min_EM_kW : Inport  Port=4
  P2 Motor : Subsystem  VariantControl=pt.P2 == 1
  P2 Motor disabled : Subsystem  VariantControl=pt.P2 == 0
  P2_M_Nm_Fahren : Outport
  P2_M_Nm_Reku : Outport  Port=2
  P_max_EM_P2_kW : Outport  Port=3
  P_min_EM_P2_kW : Outport  Port=4

== system Simulation_Fahrmodell_v3/Vehicle Dynamics Model /Drivetrain/Primary and Secondary Axle Powertrain Selector/Primary Axle Powertrain Selector/Hybrid Drive/P3 ==
  note: 1) Add Subsystem or Model blocks as valid variant choices.
      | 2) You cannot connect blocks at this level. At simulation, connectivity is automatically
      | determined, based on the active variant and port name matching.
  n_Upmin IN : Inport
  tq_sh_P3_des : Inport  Port=2
  P_max_EM_kW : Inport  Port=3
  P_min_EM_kW : Inport  Port=4
  P3 Motor : Subsystem  VariantControl=pt.P3 == 1
  P3 Motor disabled : Subsystem  VariantControl=pt.P3 == 0
  P3_M_Nm_Drive : Outport
  P3_M_Nm_Recu : Outport  Port=2
  P_max_EM_P3_kW : Outport  Port=3
  P_min_EM_P3_kW : Outport  Port=4

== system Simulation_Fahrmodell_v3/Vehicle Dynamics Model /Drivetrain/Primary and Secondary Axle Powertrain Selector/Primary Axle Powertrain Selector/Hybrid Drive/Recuperation Limit ==
  Torque_Recu_In : Inport
  Constant : Constant  Value=0
  Gain5 : Gain  Gain=100
  Recuperation Limit : Constant  Value=bat.SOC_Recup_Limit
  Relational Operator2 : RelationalOperator  Operator=<  OutDataTypeStr=boolean  RndMeth=Simplest  InputSameDT=off
  Switch2 : Switch  Criteria=u2 > Threshold  SaturateOnIntegerOverflow=off  InputSameDT=off
  Torque_Recu_Out : Outport
  wires:
  Constant/1 -> Switch2/3
  [SOC] -> Relational Operator2/1
  Recuperation Limit/1 -> Gain5/1
  Relational Operator2/1 -> Switch2/2
  Torque_Recu_In/1 -> Switch2/1
  Switch2/1 -> Torque_Recu_Out/1
  Gain5/1 -> Relational Operator2/2

== system Simulation_Fahrmodell_v3/Vehicle Dynamics Model /Drivetrain/Primary and Secondary Axle Powertrain Selector/Primary Axle Powertrain Selector/Hybrid Drive/Recuperation Limit1 ==
  Torque_Recu_In : Inport
  Constant : Constant  Value=0
  Gain5 : Gain  Gain=100
  Recuperation Limit : Constant  Value=bat.SOC_Recup_Limit
  Relational Operator2 : RelationalOperator  Operator=<  OutDataTypeStr=boolean  RndMeth=Simplest  InputSameDT=off
  Switch2 : Switch  Criteria=u2 > Threshold  SaturateOnIntegerOverflow=off  InputSameDT=off
  Torque_Recu_Out : Outport
  wires:
  Constant/1 -> Switch2/3
  [SOC] -> Relational Operator2/1
  Recuperation Limit/1 -> Gain5/1
  Relational Operator2/1 -> Switch2/2
  Torque_Recu_In/1 -> Switch2/1
  Switch2/1 -> Torque_Recu_Out/1
  Gain5/1 -> Relational Operator2/2

== system Simulation_Fahrmodell_v3/Vehicle Dynamics Model /Drivetrain/Primary and Secondary Axle Powertrain Selector/Primary Axle Powertrain Selector/Hybrid Drive/Shifting Power Cut ==
  In1 : Inport
  Constant : Constant  Value=100
  Switch2 : Switch  Criteria=u2 > Threshold  SaturateOnIntegerOverflow=off  InputSameDT=off
  Out1 : Outport
  wires:
  Constant/1 -> Switch2/3
  In1/1 -> Switch2/1
  Switch2/1 -> Out1/1
  [Clutch_Engaged] -> Switch2/2

== system Simulation_Fahrmodell_v3/Vehicle Dynamics Model /Drivetrain/Primary and Secondary Axle Powertrain Selector/Primary Axle Powertrain Selector/Hybrid Drive/Shifting Power Cut1 ==
  In1 : Inport
  Constant : Constant  Value=-100
  Switch2 : Switch  Criteria=u2 > Threshold  SaturateOnIntegerOverflow=off  InputSameDT=off
  Out1 : Outport
  wires:
  [Clutch_Engaged] -> Switch2/2
  Switch2/1 -> Out1/1
  In1/1 -> Switch2/1
  Constant/1 -> Switch2/3

== system Simulation_Fahrmodell_v3/Vehicle Dynamics Model /Drivetrain/Primary and Secondary Axle Powertrain Selector/Primary Axle Powertrain Selector/Hybrid Drive/Wirkungsgrad Antriebsstrang ==
  M_Nm IN : Inport
  Constant1 : Constant  Value=0.92
  Fahren : Product
  Reku : Product  Inputs=*/
  Switch1 : Switch  Criteria=u2 > Threshold  SaturateOnIntegerOverflow=off  InputSameDT=off
  M_Nm OUT : Outport
  wires:
  Constant1/1 -> Reku/2, Fahren/2
  M_Nm IN/1 -> Switch1/2, Reku/1, Fahren/1
  Reku/1 -> Switch1/3
  Switch1/1 -> M_Nm OUT/1
  Fahren/1 -> Switch1/1

== system Simulation_Fahrmodell_v3/Vehicle Dynamics Model /Drivetrain/Primary and Secondary Axle Powertrain Selector/Secondary Axle Powertrain Selector/Auswahl P4, P4_Dual-Motor/No Secondary Axle ==
  n_mot_Upmin : Inport
  Regelfaktor1 : Inport  Port=2
  iAG : Inport  Port=3
  i_ges : Inport  Port=4
  Torque_sh : Inport  Port=5
  Constant : Constant  Value=0
  Terminator{,1..4} (5 alike) : Terminator
  M_Nm GET P4 : Outport
  wires:
  Constant/1 -> M_Nm GET P4/1
  i_ges/1 -> Terminator/1
  iAG/1 -> Terminator1/1
  Regelfaktor1/1 -> Terminator2/1
  n_mot_Upmin/1 -> Terminator3/1
  Torque_sh/1 -> Terminator4/1

== system Simulation_Fahrmodell_v3/Vehicle Dynamics Model /Drivetrain/Primary and Secondary Axle Powertrain Selector/Secondary Axle Powertrain Selector/Auswahl P4, P4_Dual-Motor/P4 // E2 Single Motor ==
  n_mot_Upmin : Inport
  Regelfaktor1 : Inport  Port=2
  iAG : Inport  Port=3
  i_ges : Inport  Port=4
  Torque_sh : Inport  Port=5
  1-D Lookup Table1 : Lookup_n-D  NumberOfTableDimensions=1  BreakpointsForDimension1=cp.speed_breakpoints_P4  Table=cp.torque_values_P4  InternalRulePriority=Speed  RndMeth=Simplest
  AG Übersetzung : Product
  Battery and Operating Strategy Limitation (Drive) : Subsystem
  Battery and Operating Strategy Limitation (Recuperation) : Subsystem
  Bus Selector : BusSelector  OutputSignals=tq_sh_P4_des
  Constant : Constant  Value=gb.i_ges_P4
  Constant1 : Constant  Value=gb.i_ges_P4
  Constant5 : Constant  Value=0
  Divide : Product  Inputs=*/
  Gain : Gain  Gain=-1
  Min : MinMax  Inputs=2
  Power Calculation : Subsystem
  "Power Calculation " : Subsystem
  Product : Product
  Relational Operator1 : RelationalOperator  OutDataTypeStr=boolean  RndMeth=Simplest  InputSameDT=off
  Saturation : Saturate  UpperLimit=inf  LowerLimit=0
  Saturation1 : Saturate  UpperLimit=inf  LowerLimit=1
  Smoothing Logic sanfterer Übergang1 : TransferFcn  Denominator=[0.17 1]
  Switch1 : Switch  Criteria=u2 > Threshold  SaturateOnIntegerOverflow=off  InputSameDT=off
  Terminator : Terminator
  M_Nm GET P4 : Outport
  tag scope: P_max_EM_P4_kW=global, P_min_EM_P4_kW=global, tq_sh_P4_max=global
  wires:
  Regelfaktor1/1 -> Relational Operator1/1  "Regelfaktor1"
  Smoothing Logic sanfterer Übergang1/1 -> AG Übersetzung/2
  Relational Operator1/1 -> Switch1/2
  Constant5/1 -> Relational Operator1/2
  Switch1/1 -> Smoothing Logic sanfterer Übergang1/1  "Gesamtmoment motorseitig"
  AG Übersetzung/1 -> M_Nm GET P4/1
  Constant/1 -> AG Übersetzung/1
  iAG/1 -> Terminator/1  "iAG"
  i_ges/1 -> Saturation1/1
  Power Calculation/1(P_kW) -> [P_max_EM_P4_kW]  "P_max_EM_P4_kW"
  Bus Selector/1 -> Saturation/1  "<tq_sh_P4_des>"
  Product/1 -> Battery and Operating Strategy Limitation (Recuperation)/1(Motordrehzahl (1/min)), Battery and Operating Strategy Limitation (Drive)/1(Motordrehzahl (1/min)), 1-D Lookup Table1/1  "Motordrehzahl (1/min)"
  Saturation/1 -> Min/2
  "Power Calculation "/1(P_kW) -> [P_min_EM_P4_kW]  "P_min_EM_P4_kW"
  1-D Lookup Table1/1 -> Gain/1, [tq_sh_P4_max], Min/1
  Torque_sh/1 -> Bus Selector/1
  n_mot_Upmin/1 -> Divide/1  "Motordrehzahl (1/min)"
  Divide/1 -> Product/1  "Motordrehzahl (1/min)"
  Constant1/1 -> Product/2
  Saturation1/1 -> Divide/2
  Battery and Operating Strategy Limitation (Drive)/2(tq_sh_P4_bat_limted) -> Switch1/1, Power Calculation/2(tq_sh_P4_bat_limted)
  Min/1 -> Battery and Operating Strategy Limitation (Drive)/2(Torque_Drive_In)
  [P_max_EM_kW] -> Battery and Operating Strategy Limitation (Drive)/3(P_max_EV_kW)  "P_max_EM_kW"
  Battery and Operating Strategy Limitation (Drive)/1(n_Upmin OUT) -> Power Calculation/1(n_Upmin)
  Battery and Operating Strategy Limitation (Recuperation)/2(tq_sh_P4_bat_limted_recu) -> Switch1/3, "Power Calculation "/2(tq_sh_P4_bat_limted_recu)
  Gain/1 -> Battery and Operating Strategy Limitation (Recuperation)/2(Torque_Recu_In)
  [P_min_EM_kW] -> Battery and Operating Strategy Limitation (Recuperation)/3(P_min_EV_kW)  "P_min_EM_kW"
  Battery and Operating Strategy Limitation (Recuperation)/1(n_Upmin OUT) -> "Power Calculation "/1(n_Upmin)

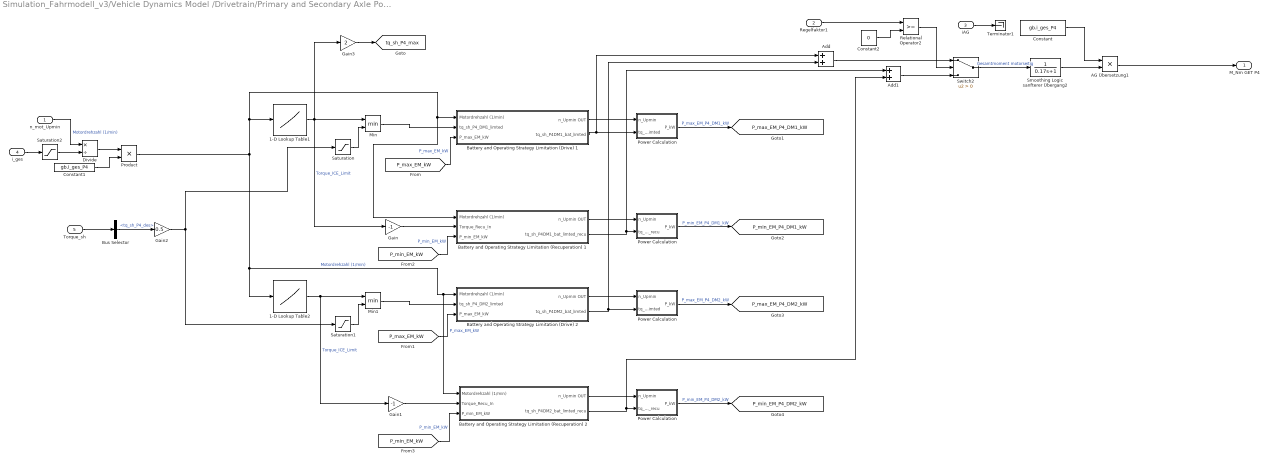
== system Simulation_Fahrmodell_v3/Vehicle Dynamics Model /Drivetrain/Primary and Secondary Axle Powertrain Selector/Secondary Axle Powertrain Selector/Auswahl P4, P4_Dual-Motor/P4 // E3 // E4 Dual Motor ==
  n_mot_Upmin : Inport
  Regelfaktor1 : Inport  Port=2
  iAG : Inport  Port=3
  i_ges : Inport  Port=4
  Torque_sh : Inport  Port=5
  1-D Lookup Table1 : Lookup_n-D  NumberOfTableDimensions=1  BreakpointsForDimension1=cp.speed_breakpoints_P4  Table=cp.torque_values_P4  InternalRulePriority=Speed  RndMeth=Simplest
  1-D Lookup Table2 : Lookup_n-D  NumberOfTableDimensions=1  BreakpointsForDimension1=cp.speed_breakpoints_P4  Table=cp.torque_values_P4  InternalRulePriority=Speed  RndMeth=Simplest
  AG Übersetzung1 : Product
  Add : Sum
  Add1 : Sum
  Battery and Operating Strategy Limitation (Drive) 1 : Subsystem
  Battery and Operating Strategy Limitation (Drive) 2 : Subsystem
  Battery and Operating Strategy Limitation (Recuperation) 1 : Subsystem
  Battery and Operating Strategy Limitation (Recuperation) 2 : Subsystem
  Bus Selector : BusSelector  OutputSignals=tq_sh_P4_des
  Constant : Constant  Value=gb.i_ges_P4
  Constant1 : Constant  Value=gb.i_ges_P4
  Constant2 : Constant  Value=0
  Divide : Product  Inputs=*/
  Gain : Gain  Gain=-1
  Gain1 : Gain  Gain=-1
  Gain2 : Gain  Gain=0.5
  Gain3 : Gain  Gain=2
  Min : MinMax  Inputs=2
  Min1 : MinMax  Inputs=2
  "Power Calculation " : Subsystem
  "Power Calculation   " : Subsystem
  "Power Calculation    " : Subsystem
  "Power Calculation     " : Subsystem
  Product : Product
  Relational Operator2 : RelationalOperator  OutDataTypeStr=boolean  RndMeth=Simplest  InputSameDT=off
  Saturation : Saturate  UpperLimit=inf  LowerLimit=0
  Saturation1 : Saturate  UpperLimit=inf  LowerLimit=0
  Saturation2 : Saturate  UpperLimit=inf  LowerLimit=1
  Smoothing Logic sanfterer Übergang2 : TransferFcn  Denominator=[0.17 1]
  Switch2 : Switch  Criteria=u2 > Threshold  SaturateOnIntegerOverflow=off  InputSameDT=off
  Terminator1 : Terminator
  M_Nm GET P4 : Outport
  tag scope: P_max_EM_P4_DM1_kW=global, P_max_EM_P4_DM2_kW=global, P_min_EM_P4_DM1_kW=global, P_min_EM_P4_DM2_kW=global, tq_sh_P4_max=global
  wires:
  Bus Selector/1 -> Gain2/1  "<tq_sh_P4_des>"
  "Power Calculation    "/1(P_kW) -> [P_min_EM_P4_DM1_kW]  "P_min_EM_P4_DM1_kW"
  Torque_sh/1 -> Bus Selector/1
  "Power Calculation     "/1(P_kW) -> [P_max_EM_P4_DM1_kW]  "P_max_EM_P4_DM1_kW"
  1-D Lookup Table1/1 -> Gain3/1, Min/1, Gain/1  "Torque_ICE_Limit"
  Saturation/1 -> Min/2
  "Power Calculation "/1(P_kW) -> [P_min_EM_P4_DM2_kW]  "P_min_EM_P4_DM2_kW"
  "Power Calculation   "/1(P_kW) -> [P_max_EM_P4_DM2_kW]  "P_max_EM_P4_DM2_kW"
  1-D Lookup Table2/1 -> Gain1/1, Min1/1  "Torque_ICE_Limit"
  Saturation1/1 -> Min1/2
  AG Übersetzung1/1 -> M_Nm GET P4/1
  Constant/1 -> AG Übersetzung1/1
  Switch2/1 -> Smoothing Logic sanfterer Übergang2/1  "Gesamtmoment motorseitig"
  iAG/1 -> Terminator1/1
  Relational Operator2/1 -> Switch2/2
  Regelfaktor1/1 -> Relational Operator2/1
  Add1/1 -> Switch2/3
  Constant2/1 -> Relational Operator2/2
  Add/1 -> Switch2/1
  Smoothing Logic sanfterer Übergang2/1 -> AG Übersetzung1/2
  Gain2/1 -> Saturation/1, Saturation1/1
  n_mot_Upmin/1 -> Divide/1  "Motordrehzahl (1/min)"
  i_ges/1 -> Saturation2/1
  Divide/1 -> Product/1
  Constant1/1 -> Product/2
  Product/1 -> Battery and Operating Strategy Limitation (Recuperation) 1/1(Motordrehzahl (1/min)), Battery and Operating Strategy Limitation (Drive) 1/1(Motordrehzahl (1/min)), 1-D Lookup Table1/1, 1-D Lookup Table2/1, Battery and Operating Strategy Limitation (Recuperation) 2/1(Motordrehzahl (1/min)), Battery and Operating Strategy Limitation (Drive) 2/1(Motordrehzahl (1/min))  "Motordrehzahl (1/min)"
  Saturation2/1 -> Divide/2
  Gain3/1 -> [tq_sh_P4_max]
  Battery and Operating Strategy Limitation (Drive) 1/2(tq_sh_P4DM1_bat_limted) -> Add/1, "Power Calculation     "/2(tq_sh_P4DM1_bat_limted)
  Min/1 -> Battery and Operating Strategy Limitation (Drive) 1/2(tq_sh_P4_DM1_limted)
  [P_max_EM_kW] -> Battery and Operating Strategy Limitation (Drive) 1/3(P_max_EM_kW)  "P_max_EM_kW"
  Battery and Operating Strategy Limitation (Drive) 1/1(n_Upmin OUT) -> "Power Calculation     "/1(n_Upmin)
  Battery and Operating Strategy Limitation (Recuperation) 1/2(tq_sh_P4DM1_bat_limted_recu) -> Add1/1, "Power Calculation    "/2(tq_sh_P4DM1_bat_limted_recu)
  Gain/1 -> Battery and Operating Strategy Limitation (Recuperation) 1/2(Torque_Recu_In)
  [P_min_EM_kW] -> Battery and Operating Strategy Limitation (Recuperation) 1/3(P_min_EM_kW)  "P_min_EM_kW"
  Battery and Operating Strategy Limitation (Recuperation) 1/1(n_Upmin OUT) -> "Power Calculation    "/1(n_Upmin)
  Battery and Operating Strategy Limitation (Drive) 2/2(tq_sh_P4DM2_bat_limted) -> Add/2, "Power Calculation   "/2(tq_sh_P4DM2_bat_limted)
  Min1/1 -> Battery and Operating Strategy Limitation (Drive) 2/2(tq_sh_P4_DM2_limted)
  [P_max_EM_kW] -> Battery and Operating Strategy Limitation (Drive) 2/3(P_max_EM_kW)  "P_max_EM_kW"
  Battery and Operating Strategy Limitation (Drive) 2/1(n_Upmin OUT) -> "Power Calculation   "/1(n_Upmin)
  Battery and Operating Strategy Limitation (Recuperation) 2/2(tq_sh_P4DM2_bat_limted_recu) -> Add1/2, "Power Calculation "/2(tq_sh_P4DM2_bat_limted_recu)
  Gain1/1 -> Battery and Operating Strategy Limitation (Recuperation) 2/2(Torque_Recu_In)
  [P_min_EM_kW] -> Battery and Operating Strategy Limitation (Recuperation) 2/3(P_min_EM_kW)  "P_min_EM_kW"
  Battery and Operating Strategy Limitation (Recuperation) 2/1(n_Upmin OUT) -> "Power Calculation "/1(n_Upmin)
